simulink model "BLDC1"  (R2012b)
settings: Solver=ode45  StartTime=0.0  StopTime=3  RelTol=1e-3
libraries: BLDC x2
settings Model: Creator=h3now  LastModifiedBy=h3now

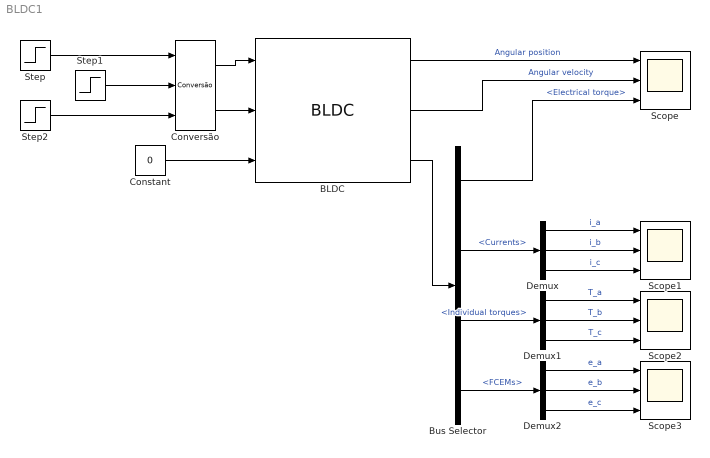
== system BLDC1 ==
  BLDC : BLDC/BLDC  J=1.39e-6  R=10.1/2  L=2.04/2000  P=8  Kt=15.7e-3/1.19  Ke=15.7e-3/1.19  Kd=0  F_stick=0  F_slip=0  default_fcem=on  fcem_a=fcem_a  fcem_b=fcem_b  fcem_c=fcem_c
  Bus Selector : BusSelector  OutputSignals=Electrical torque,Currents,Individual torques,FCEMs
  Constant : Constant  Value=0
  Conversão : BLDC/Conversão
  Demux : Demux  Outputs=3
  Demux1 : Demux  Outputs=3
  Demux2 : Demux  Outputs=3
  Scope{,1..3} (4 alike) : Scope  NumInputPorts=3
      Scope settings: ShowLegends=on  YMin=-5~-5~-5  YMax=5~5~5
      Scope1 settings: YMin=-5~-5~-5  YMax=5~5~5
      Scope2 settings: YMin=-5~-5~-5  YMax=5~5~5  SaveName=ScopeData2
      Scope3 settings: YMin=-5~-5~-5  YMax=5~5~5  SaveName=ScopeData3
  Step : Step  Time=0  Before=20  After=20  SampleTime=0
  Step1 : Step  After=20  SampleTime=0
  Step2 : Step  Time=2  After=20  SampleTime=0
  wires:
  BLDC/1 -> Scope/1  "Angular position"
  BLDC/2 -> Scope/2  "Angular velocity"
  BLDC/3 -> Bus Selector/1
  Bus Selector/1 -> Scope/3  "<Electrical torque>"
  Bus Selector/2 -> Demux/1  "<Currents>"
  Bus Selector/3 -> Demux1/1  "<Individual torques>"
  Bus Selector/4 -> Demux2/1  "<FCEMs>"
  Demux/1 -> Scope1/1  "i_a"
  Demux/2 -> Scope1/2  "i_b"
  Demux/3 -> Scope1/3  "i_c"
  Demux1/1 -> Scope2/1  "T_a"
  Demux1/2 -> Scope2/2  "T_b"
  Demux1/3 -> Scope2/3  "T_c"
  Demux2/1 -> Scope3/1  "e_a"
  Demux2/2 -> Scope3/2  "e_b"
  Demux2/3 -> Scope3/3  "e_c"
  Conversão/1 -> BLDC/1
  Conversão/2 -> BLDC/2
  Step1/1 -> Conversão/2
  Step/1 -> Conversão/1
  Step2/1 -> Conversão/3
  Constant/1 -> BLDC/3
